simulink model "Vespula_HIiLo_Control"  (R2025b)
settings: Solver=VariableStepAuto  StartTime=0.0  StopTime=30.0  RelTol=1e-3
InitFcn:
  | load('FuelPropsData.mat')
libraries: fl_lib x33, nesl_utility x27, SimscapeFluids_lib x10
(part 1 of 3)
settings Model: Creator=mbdal  LastModifiedBy=25han
settings SolverCC: MaxConsecutiveMinStep=100  ZeroCrossAlgorithm=Adaptive
settings OptimizationCC: ReuseModelBlockBuffer=off
settings DebuggingCC: IgnoredZcDiagnostic=none
settings RTWCC: GPUComputeCapability=3.5

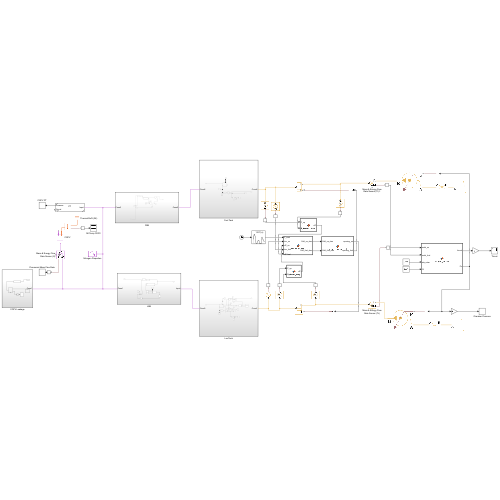
[thumbnail: Simulink's stored preview of the top-level diagram]
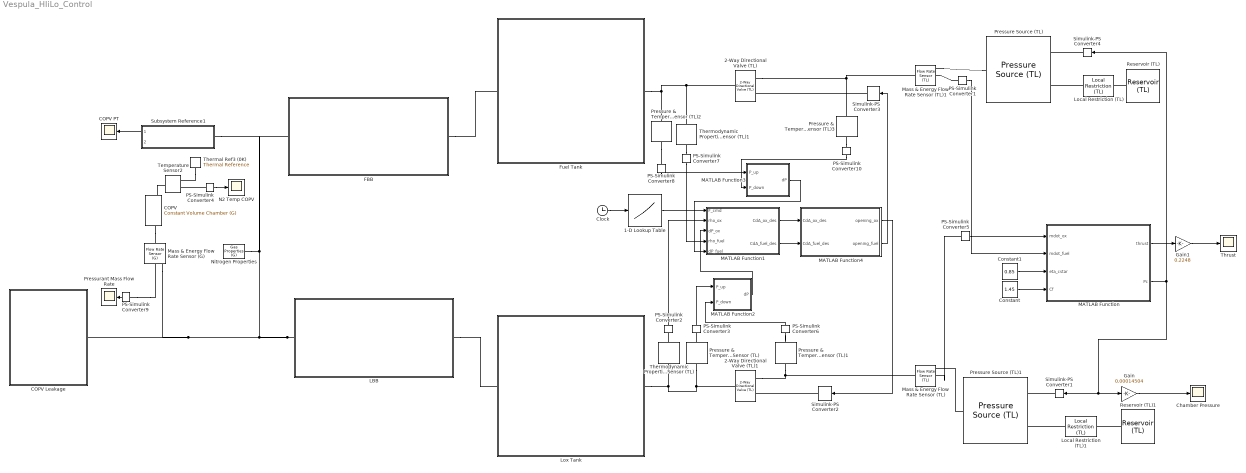
== system Vespula_HIiLo_Control ==
  1-D Lookup Table : Lookup_n-D  NumberOfTableDimensions=1  BreakpointsForDimension1=|  Table=|  InternalRulePriority=Speed  RndMeth=Simplest
      BreakpointsForDimension1=|
      | [0
      | 2.46e-15
      | 4.93e-15
      | 1.31e-14
      | 1.85798e-4
      | 3.71595e-4
      | 1.300583e-3
      | 5.945524e-3
      | 2.917023e-2
      | 1.452937e-1
      | 3.251823e-1
      | 6.176896e-1
      | 1.048884
      | 1.648122
      | 2.452841
      | 3.452841
      | 4.452841
      | 5.452841
      | 6.452841
      | 7.452841
      | 8.452841
      | 9.452841
      | 10.45284
      | 11.45284
      | 12.45284
      | 13.45284
      | 14.45284
      | 15.45284
      | 16.26888
      | 17.26888
      | 18.26888
      | 19.26888
      | 20.26888
      | 21.26888
      | 21.82014
      | 22.37140
      | 23.10183
      | 24.10183
      | 25.10183
      | 26.10183
      | 27.10183
      | 28.10183
      | 29.10183
      | 29.70287]
      Table=|
      | [1115.929794
      | 1115.929794
      | 1115.929794
      | 1115.929794
      | 1116.015031
      | 1116.100248
      | 1116.526042
      | 1118.647732
      | 1129.075722
      | 1176.888468
      | 1237.984070
      | 1309.087819
      | 1365.657208
      | 1382.500173
      | 1347.869214
      | 1276.732855
      | 1209.886660
      | 1007.359221
      | 890.000000
      | 890.000000
      | 890.000000
      | 890.000000
      | 970.372958
      | 1015.368113
      | 1034.720854
      | 1040.888013
      | 1040.596927
      | 896.870767
      | 890.000000
      | 890.000000
      | 890.000000
      | 890.000000
      | 890.000000
      | 890.000000
      | 1074.062231
      | 1213.486737
      | 1218.338865
      | 1172.384789
      | 1114.978943
      | 1066.195681
      | 1030.043331
      | 1004.841448
      | 987.599936
      | 979.912878]
  2-Way Directional Valve (TL) : SimscapeFluids_lib/Thermal Liquid/Valves & Orifices/Directional Control Valves/2-Way Directional Valve (TL)  valve_spec=fluids.thermal_liquid.valves.directional_control_valves.enum.ValveSpec.Table1DAreaOpening  S_max=1 m  del_S_max=5e-3 m  area_max=1e-4 m^2  area_leak=1e-10 m^2  del_S_TLU=[0 0.3 0.4 0.5 0.6 0.7 0.8 0.9 1.0] m  valve_area_TLU=[1e-9 1.7065e-07 1.0239e-06 3.5836e-06 7.8498e-06 1.4164e-05 2.3038e-05 3.4812e-05 5.0000e-05] m^2  del_S_flow_TLU=[0, .002, .004, .007, .017] m  p_diff_TLU=[.3, .5, .7] MPa  vol_flow_TLU=1e-3 * [1.7e-05, 2e-05, 2.6e-05; .0035, .0045, .0053; .7, .9, 1.06; 1.96, 2.5, 3; 6, 7.7, 9.13] m^3/s  mdot_TLU=[1.7e-05, 2e-05, 2.6e-05; .0035, .0045, .0053; .7, .9, 1.06; 1.96, 2.5, 3; 6, 7.7, 9.13] kg/s  T_ref_in=293.15 K  p_ref_in=0.101325 MPa  Cd=1  Re_c=150  smoothing_factor=0.01  pressure_recovery=false  area=0.01 m^2
      settings: InternalSimscapePortConfiguration="{\"Bottom\":[],\"Left\":[{\"id\":\"A\",\"label\":\"A\",\"type\":\"foundation.thermal_liquid.thermal_liquid\"}],\"Right\":[{\"id\":\"S\",\"label\":\"S\",\"type\":\"input\"},{\"id\":\"B\",\"label\":\"B\",\"type\":\"foundation.thermal_liquid.thermal_liquid\"}],\"Top\":[]}"
  2-Way Directional Valve (TL)1 : SimscapeFluids_lib/Thermal Liquid/Valves & Orifices/Directional Control Valves/2-Way Directional Valve (TL)  valve_spec=fluids.thermal_liquid.valves.directional_control_valves.enum.ValveSpec.Table1DAreaOpening  S_max=1 m  del_S_max=5e-3 m  area_max=1e-4 m^2  area_leak=1e-10 m^2  del_S_TLU=[0 0.3 0.4 0.5 0.6 0.7 0.8 0.9 1.0] m  valve_area_TLU=[1e-9 1.7065e-07 1.0239e-06 3.5836e-06 7.8498e-06 1.4164e-05 2.3038e-05 3.4812e-05 5.0000e-05] m^2  del_S_flow_TLU=[0, .002, .004, .007, .017] m  p_diff_TLU=[.3, .5, .7] MPa  vol_flow_TLU=1e-3 * [1.7e-05, 2e-05, 2.6e-05; .0035, .0045, .0053; .7, .9, 1.06; 1.96, 2.5, 3; 6, 7.7, 9.13] m^3/s  mdot_TLU=[1.7e-05, 2e-05, 2.6e-05; .0035, .0045, .0053; .7, .9, 1.06; 1.96, 2.5, 3; 6, 7.7, 9.13] kg/s  T_ref_in=293.15 K  p_ref_in=0.101325 MPa  Cd=1  Re_c=150  smoothing_factor=0.01  pressure_recovery=false  area=0.01 m^2
      settings: InternalSimscapePortConfiguration="{\"Bottom\":[],\"Left\":[{\"id\":\"A\",\"label\":\"A\",\"type\":\"foundation.thermal_liquid.thermal_liquid\"}],\"Right\":[{\"id\":\"S\",\"label\":\"S\",\"type\":\"input\"},{\"id\":\"B\",\"label\":\"B\",\"type\":\"foundation.thermal_liquid.thermal_liquid\"}],\"Top\":[]}"
  COPV : fl_lib/Gas/Elements/Constant Volume Chamber (G)  volume=18 l  num_ports=foundation.enum.num_ports.two  area_A=0.01 m^2  area_B=0.8 in^2  area_C=0.01 m^2  area_D=0.01 m^2  p_I_specify=on  p_I_priority=Low  p_I=4500 psi  p_I_nominal_specify=off  p_I_nominal_value=1  p_I_nominal_unit=MPa  T_I_specify=on  T_I_priority=Low  T_I=60 degF  T_I_nominal_specify=off  T_I_nominal_value=1  T_I_nominal_unit=K  rho_I_specify=off  rho_I_priority=None  rho_I=1.2 kg/m^3  rho_I_nominal_specify=off  rho_I_nominal_value=1  rho_I_nominal_unit=kg/m^3
      settings: InternalSimscapePortConfiguration="{\"Bottom\":[],\"Left\":[{\"id\":\"A\",\"label\":\"A\",\"type\":\"foundation.gas.gas\"},{\"id\":\"H\",\"label\":\"H\",\"type\":\"foundation.thermal.thermal\"}],\"Right\":[{\"id\":\"B\",\"label\":\"B\",\"type\":\"foundation.gas.gas\"}],\"Top\":[]}"
  COPV Leakage : Subsystem
  COPV PT : Scope
      settings: ActiveDisplayYMinimum=1666.95319727996  ActiveDisplayYMaximum=5313.5498863404391  DataLoggingVariableName=ScopeData4  DataLoggingSaveFormat=Array
  Chamber Pressure : Scope
      settings: ActiveDisplayYMinimum=-162.39251881911565  ActiveDisplayYMaximum=515.77790198606317  DataLoggingVariableName=ScopeData22
  Clock : Clock
  Constant : Constant  Value=1.45
  Constant1 : Constant  Value=0.85
  FBB : Subsystem
  Fuel Tank : Subsystem
  Gain : Gain  Gain=0.00014504
  Gain1 : Gain  Gain=0.2248
  LBB : Subsystem
  Local Restriction (TL) : fl_lib/Thermal Liquid/Elements/Local Restriction (TL)  restriction_type=foundation.enum.restriction_type.fixed  restriction_area=0.001 m^2  min_area=1e-10 m^2  max_area=0.005 m^2  area=0.01 m^2  Cd=0.64  Re_c=150  pressure_recovery=true
  Local Restriction (TL)1 : fl_lib/Thermal Liquid/Elements/Local Restriction (TL)  restriction_type=foundation.enum.restriction_type.fixed  restriction_area=0.001 m^2  min_area=1e-10 m^2  max_area=0.005 m^2  area=0.01 m^2  Cd=0.64  Re_c=150  pressure_recovery=true
  Lox Tank : Subsystem
  MATLAB Function : MATLAB Function  TreatAsAtomicUnit=on
  MATLAB Function1 : MATLAB Function  TreatAsAtomicUnit=on
  MATLAB Function2 : MATLAB Function  TreatAsAtomicUnit=on
  MATLAB Function3 : MATLAB Function  TreatAsAtomicUnit=on
  MATLAB Function4 : MATLAB Function  TreatAsAtomicUnit=on
  Mass & Energy Flow Rate Sensor (G) : fl_lib/Gas/Sensors/Flow Rate Sensor (G)  mass_flow_measure=true  volumetric_flow_measure=false  volumetric_flow_conditions=foundation.enum.volumetric_flow_conditions.actual  p_std=0.101325 MPa  T_std=20 degC  energy_flow_measure=true
      settings: InternalSimscapePortConfiguration="{\"Bottom\":[{\"id\":\"PHI\",\"label\":\"φ\",\"type\":\"output\"}],\"Left\":[{\"id\":\"A\",\"label\":\"A\",\"type\":\"foundation.gas.gas\"}],\"Right\":[{\"id\":\"B\",\"label\":\"B\",\"type\":\"foundation.gas.gas\"},{\"id\":\"M\",\"label\":\"M\",\"type\":\"output\"}],\"Top\":[]}"
  Mass & Energy Flow Rate Sensor (TL) : fl_lib/Thermal Liquid/Sensors/Flow Rate Sensor (TL)  mass_flow_measure=true  volumetric_flow_measure=false  energy_flow_measure=true
      settings: InternalSimscapePortConfiguration="{\"Bottom\":[{\"id\":\"PHI\",\"label\":\"φ\",\"type\":\"output\"}],\"Left\":[{\"id\":\"A\",\"label\":\"A\",\"type\":\"foundation.thermal_liquid.thermal_liquid\"}],\"Right\":[{\"id\":\"B\",\"label\":\"B\",\"type\":\"foundation.thermal_liquid.thermal_liquid\"},{\"id\":\"M\",\"label\":\"M\",\"type\":\"output\"}],\"Top\":[]}"
  Mass & Energy Flow Rate Sensor (TL)1 : fl_lib/Thermal Liquid/Sensors/Flow Rate Sensor (TL)  mass_flow_measure=true  volumetric_flow_measure=false  energy_flow_measure=true
      settings: InternalSimscapePortConfiguration="{\"Bottom\":[{\"id\":\"PHI\",\"label\":\"φ\",\"type\":\"output\"}],\"Left\":[{\"id\":\"A\",\"label\":\"A\",\"type\":\"foundation.thermal_liquid.thermal_liquid\"}],\"Right\":[{\"id\":\"B\",\"label\":\"B\",\"type\":\"foundation.thermal_liquid.thermal_liquid\"},{\"id\":\"M\",\"label\":\"M\",\"type\":\"output\"}],\"Top\":[]}"
  N2 Temp COPV : Scope
      settings: ActiveDisplayYMinimum=266.75436250244837  ActiveDisplayYMaximum=294.5410897859407  DataLoggingVariableName=ScopeData11
  Nitrogen Properties : fl_lib/Gas/Utilities/Gas Properties (G)  gas_spec=foundation.enum.gas_spec.real_gas  R=0.297 kJ/(K*kg)  Z=1  T_ref=293.0 K  h_ref=425.45 kJ/kg  cp_ref=1.1305 kJ/(K*kg)  mu_ref=24.664 s*uPa  k_ref=24.664 W/(m*K)  T_TLU1=[150 : 10 : 200, 250 : 50 : 1000, 1500, 2000]' K  h_TLU1=[275.264783730547; 285.377054177734; 295.474578903607; 305.560871069627; 315.638490783961; 325.709373787179; 376.008033649461; 426.297784741196; 476.678788323875; 527.253890684429; 578.12722735187; 629.395040865183; 681.137690131207; 733.415442873049; 786.267894376777; 839.715851152006; 893.764459999509; 948.406676876931; 1003.62653219711; 1059.40193232821; 1115.70691941005; 1172.51341226958; 1762.18512007361; 2377.14064127409] kJ/kg  cp_TLU1=[1.01211492398124; 1.01042105529234; 1.00914159006373; 1.00815898273273; 1.00739688341918; 1.00680484569075; 1.00554191216852; 1.00637389921747; 1.0092105862442; 1.01414404435034; 1.02111299587909; 1.02986878923959; 1.04003820504128; 1.05120320041448; 1.06296312852444; 1.07497111709439; 1.08694865668905; 1.0986858495625; 1.11003396604319; 1.12089493621399; 1.13121051694521; 1.14095251451866; 1.21001953144; 1.24628356718428] kJ/(K*kg)  mu_TLU1=[10.3766056544352; 10.9908682444892; 11.5932000841352; 12.1841060353213; 12.764067709023; 13.3335437107148; 16.038149065057; 18.5373404836509; 20.8671495114253; 23.0554226800681; 25.1239717991959; 27.0901379793485; 28.96790749834; 30.7687111230031; 32.5020036481173; 34.17569027566; 35.7964450415303; 37.3699520751368; 38.9010908824946; 40.3940804368247; 41.8525925389218; 43.279841956487; 56.3254722619962; 68.068290080945] s*uPa  k_TLU1=[14.1517155766309; 15.0474512994325; 15.9300520513026; 16.7998749295306; 17.6573089963228; 18.5027588910197; 22.5644026699512; 26.384465676638; 30.0032801168886; 33.4532006033488; 36.7600619429332; 39.9446251241844; 43.0237448740114; 46.0112537033799; 48.9186234516389; 51.7554617696538; 54.5298878921773; 57.2488200454925; 59.9181976996146; 62.5431553064749; 65.128159527924; 67.6771186900213; 91.7815514375552; 114.486299090693] mW/(K*m)  T_TLU2=[ 150 160 170 180 190 200 250 300 350 400 450 500 550 600 650 700 750 800 850 900 950 1000 1500 2000 ] K  p_TLU2=[ 0.001 0.005 0.01 0.02 0.03 0.04 0.05 0.06 0.07 0.08 0.09 0.1 0.12 0.15 0.2 0.5 1 2 5 10 15 20 25 30 35 ] MPa  rho_TLU2=|  s_TLU2=|  h_TLU2=|  cp_TLU2=|  mu_TLU2=|  k_TLU2=|  beta_TLU2=|  alpha_TLU2=|  T_min_perfect=1 K  T_max_perfect=inf K  p_min_perfect=1 Pa  p_max_perfect=inf MPa  T_range_flag=foundation.enum.T_range_G.from_props  T_min_semiperfect=150 K  T_max_semiperfect=2000 K  p_min_semiperfect=1 Pa  p_max_semiperfect=inf MPa  pT_region_flag=foundation.enum.pT_region_G.from_props  pT_validity_TLU2=ones(24, 20)  T_min_real=150 K  T_max_real=2000 K  p_min_real=0.001 MPa  p_max_real=10 MPa  p_atm=0.101325 MPa  properties_range_check=simscape.enum.assert.action.error  Mach_rev=0.001
      rho_TLU2=|
      | [
      |   0.0224628 0.11234 0.224745 0.449748 0.675012 0.900536 1.12632 1.35237 1.57868 1.80525 2.03209 2.25919 2.71419 3.39869 4.54491 11.5684 23.876 51.1797 168.905 419.166 512.081 561.75 596.092 622.603 644.346
      |   0.0210587 0.105313 0.210675 0.421548 0.632619 0.843889 1.05536 1.26702 1.47889 1.69096 1.90322 2.11569 2.54123 3.18105 4.25149 10.7835 22.111 46.6336 140.444 344.171 458.334 518.814 559.223 589.665 614.197
      |   0.0198197 0.0991139 0.198266 0.396684 0.595255 0.793978 0.992854 1.19188 1.39107 1.5904 1.78989 1.98953 2.38928 2.99007 3.99448 10.104 20.6157 42.9807 122.906 287.979 407.95 477.264 523.326 557.57 584.838
      |   0.0187185 0.0936044 0.187238 0.374595 0.56207 0.749663 0.937375 1.12521 1.31315 1.50122 1.68941 1.87772 2.25469 2.82104 3.76735 9.50897 19.3276 39.9514 110.475 248.744 363.904 438.437 489.087 526.714 556.514
      |   0.0177332 0.0886754 0.177374 0.35484 0.532399 0.71005 0.887794 1.06563 1.24356 1.42158 1.59969 1.7779 2.13459 2.67033 3.56509 8.98291 18.2034 37.3816 100.976 220.597 327.193 403.291 457.086 497.451 529.453
      |   0.0168465 0.0842398 0.168498 0.337068 0.50571 0.674425 0.843213 1.01207 1.18101 1.35001 1.51909 1.68824 2.02676 2.53508 3.38374 8.51404 17.2116 35.1639 93.3657 199.439 297.167 372.228 427.691 470.049 503.836
      |   0.013477 0.0673872 0.13478 0.269581 0.404403 0.539247 0.674112 0.808998 0.943905 1.07883 1.21378 1.34875 1.61876 2.02392 2.69962 6.76469 13.5801 27.3519 69.5435 140.592 208.08 268.096 319.417 362.758 399.494
      |   0.0112308 0.0561543 0.11231 0.224623 0.336941 0.449263 0.561589 0.673919 0.786253 0.898591 1.01093 1.12328 1.34798 1.68507 2.24695 5.6202 11.2488 22.5234 56.3445 111.725 164.239 212.537 256.035 294.781 329.184
      |   0.00962635 0.0481315 0.0962625 0.192523 0.288781 0.385036 0.48129 0.577541 0.67379 0.770036 0.86628 0.962522 1.155 1.44369 1.92481 4.81016 9.61356 19.1957 47.6684 93.741 137.378 178.031 215.461 249.68 280.866
      |   0.00842305 0.0421148 0.0842284 0.168452 0.252671 0.336886 0.421096 0.505301 0.589502 0.673698 0.757889 0.842076 1.01043 1.26294 1.68369 4.20567 8.39918 16.7473 41.4399 81.1856 118.842 154.174 187.094 217.632 245.899
      |   0.00748715 0.0374352 0.0748691 0.149733 0.224591 0.299444 0.374292 0.449134 0.523971 0.598803 0.673629 0.74845 0.898076 1.12247 1.49637 3.73687 7.46006 14.8641 36.7155 71.8128 105.105 136.495 165.968 193.564 219.367
      |   0.00673843 0.0336916 0.0673819 0.134758 0.20213 0.269495 0.336856 0.404211 0.47156 0.538905 0.606244 0.673577 0.808228 1.01016 1.34662 3.36249 6.71139 13.3677 32.9929 64.4976 94.4306 122.764 149.512 174.722 198.464
      |   0.00612584 0.0306287 0.0612561 0.122507 0.183753 0.244994 0.30623 0.36746 0.428686 0.489906 0.551121 0.612331 0.734736 0.918305 1.22415 3.05653 6.10019 12.1485 29.9758 58.6032 85.8531 111.73 136.264 159.502 181.505
      |   0.00561536 0.0280763 0.0561514 0.112298 0.16844 0.224577 0.28071 0.336837 0.39296 0.449078 0.505192 0.561301 0.673504 0.841773 1.12213 2.80175 5.59158 11.1353 27.4767 53.7382 78.7843 102.636 125.328 146.908 167.426
      |   0.00518341 0.0259166 0.0518321 0.10366 0.155483 0.207302 0.259117 0.310927 0.362733 0.414535 0.466332 0.518125 0.621697 0.777024 1.03581 2.58626 5.1616 10.2795 25.37 49.6461 72.8431 94.9893 116.122 136.283 155.52
      |   0.00481316 0.0240654 0.0481298 0.0962557 0.144378 0.192495 0.240609 0.288719 0.336825 0.384927 0.433025 0.481119 0.577295 0.721529 0.96184 2.40161 4.79327 9.54671 23.5687 46.1513 67.7704 88.4569 108.247 127.18 145.298
      |   0.00449229 0.0224611 0.0449212 0.0898388 0.134753 0.179663 0.22457 0.269473 0.314372 0.359268 0.40416 0.449049 0.538815 0.673437 0.897734 2.24161 4.47416 8.91208 22.0097 43.1286 63.3825 82.8028 101.424 119.282 136.413
      |   0.00421152 0.0210573 0.0421137 0.0842241 0.126331 0.168435 0.210535 0.252632 0.294726 0.336817 0.378904 0.420988 0.505146 0.631358 0.841645 2.10163 4.195 8.357 20.6467 40.4863 59.5457 77.8551 95.4466 112.353 128.607
      |   0.00396378 0.0198186 0.0396365 0.0792699 0.1189 0.158528 0.198152 0.237773 0.277392 0.317007 0.356619 0.396229 0.475438 0.59423 0.792155 1.97812 3.9487 7.86733 19.4444 38.1554 56.1594 73.485 90.1619 106.22 121.688
      |   0.00374357 0.0187176 0.0374345 0.0748662 0.112295 0.149721 0.187145 0.224565 0.261983 0.299398 0.336811 0.37422 0.449031 0.561227 0.748164 1.86834 3.72979 7.43208 18.3758 36.083 53.1469 69.5942 85.4522 100.748 115.507
      |   0.00354654 0.0177325 0.0354643 0.070926 0.106385 0.141842 0.177296 0.212748 0.248197 0.283643 0.319087 0.354529 0.425404 0.531698 0.708804 1.77011 3.53391 7.04264 17.4195 34.2275 50.4481 66.1058 81.2256 95.8317 109.948
      |   0.00336922 0.0168458 0.0336911 0.0673799 0.101066 0.13475 0.168432 0.202112 0.235789 0.269464 0.303136 0.336806 0.40414 0.505122 0.67338 1.68171 3.35761 6.69211 16.5585 32.5562 48.0155 62.959 77.4094 91.3888 104.918
      |   0.00224615 0.0112306 0.022461 0.0449208 0.0673795 0.0898371 0.112294 0.134749 0.157203 0.179656 0.202108 0.224559 0.269457 0.336796 0.449005 1.12167 2.24054 4.46991 11.0918 21.9124 32.4719 42.7798 52.8458 62.6786 72.2871
      |   0.00168461 0.00842299 0.0168458 0.033691 0.0505355 0.0673794 0.0842226 0.101065 0.117907 0.134748 0.151589 0.168429 0.202107 0.25262 0.336794 0.841502 1.6814 3.35638 8.34329 16.5303 24.5658 32.4546 40.2011 47.8097 55.2845
      | ] kg/m^3
      s_TLU2=|
      | [
      |   7.49285 7.01501 6.8091 6.603 6.48229 6.39654 6.32994 6.27546 6.22933 6.18933 6.154 6.12236 6.0675 6.00016 5.9129 5.62948 5.40371 5.15375 4.7005 4.22784 4.07775 3.99456 3.93507 3.88788 3.84829
      |   7.55991 7.08209 6.87621 6.67017 6.54951 6.46381 6.39727 6.34284 6.29678 6.25683 6.22156 6.18997 6.13523 6.06805 5.98109 5.69949 5.4771 5.23565 4.83347 4.40808 4.22227 4.12381 4.05631 4.00418 3.96125
      |   7.6229 7.1451 6.93924 6.73324 6.61263 6.52698 6.46048 6.4061 6.36008 6.32017 6.28495 6.2534 6.19875 6.13171 6.04497 5.76478 5.54497 5.30962 4.93669 4.55875 4.35631 4.24459 4.1695 4.1126 4.06642
      |   7.68229 7.20451 6.99867 6.7927 6.67213 6.58651 6.52005 6.4657 6.41971 6.37985 6.34465 6.31315 6.25857 6.19163 6.10508 5.82601 5.60821 5.37744 5.02371 4.6809 4.47723 4.35635 4.27486 4.21367 4.16448
      |   7.73847 7.2607 7.05487 6.84894 6.72839 6.6428 6.57637 6.52205 6.47609 6.43626 6.40109 6.36962 6.31509 6.24825 6.16184 5.88369 5.66748 5.44026 5.10015 4.78242 4.58443 4.45885 4.37256 4.30779 4.25597
      |   7.79177 7.31401 7.10819 6.90228 6.78176 6.69619 6.62978 6.57549 6.52956 6.48974 6.45461 6.42315 6.36868 6.30191 6.21562 5.93821 5.72331 5.4989 5.16896 4.86953 4.67917 4.55232 4.46291 4.39539 4.34139
      |   8.02365 7.54592 7.34014 7.1343 7.01386 6.92836 6.86203 6.80781 6.76195 6.72222 6.68715 6.65577 6.60145 6.5349 6.44899 6.17388 5.96289 5.74667 5.44372 5.18996 5.02917 4.9123 4.82264 4.75128 4.69272
      |   8.21316 7.73544 7.52968 7.32388 7.20347 7.11802 7.05172 6.99754 6.95172 6.91202 6.87699 6.84565 6.7914 6.72497 6.63924 6.36524 6.15613 5.94369 5.65221 5.41654 5.27019 5.16301 5.0789 5.01026 4.95271
      |   8.37353 7.89582 7.69007 7.48429 7.3639 7.27847 7.21219 7.15803 7.11223 7.07255 7.03754 7.00622 6.95202 6.88564 6.80002 6.52665 6.31857 6.10821 5.82285 5.59656 5.45806 5.35694 5.27722 5.21162 5.15607
      |   8.51273 8.03503 7.82928 7.62352 7.50314 7.41772 7.35146 7.29731 7.25152 7.21185 7.17686 7.14555 7.09137 7.02504 6.93948 6.66649 6.45906 6.24996 5.96826 5.74757 5.61385 5.51664 5.44002 5.3768 5.32307
      |   8.63597 8.15828 7.95253 7.74678 7.62641 7.541 7.47474 7.4206 7.37482 7.33516 7.30018 7.26888 7.21472 7.14841 7.06289 6.79016 6.58314 6.37487 6.09556 5.87849 5.74792 5.65337 5.57895 5.51753 5.46526
      |   8.74684 8.26914 8.06341 7.85766 7.73729 7.65189 7.58564 7.5315 7.48573 7.44608 7.4111 7.37981 7.32565 7.25936 7.17388 6.90131 6.69459 6.48688 6.20922 5.99465 5.86627 5.7736 5.70079 5.64074 5.58961
      |   8.84788 8.37018 8.16445 7.9587 7.83834 7.75294 7.68669 7.63256 7.5868 7.54715 7.51217 7.48089 7.42674 7.36046 7.275 7.00256 6.79604 6.58874 6.31225 6.09947 5.97268 5.88141 5.80981 5.7508 5.70057
      |   8.94094 8.46325 8.25751 8.05177 7.93141 7.84602 7.77977 7.72565 7.67988 7.64024 7.60526 7.57398 7.51984 7.45357 7.36812 7.09578 6.88941 6.68241 6.40679 6.19534 6.06974 5.97952 5.90885 5.85065 5.80114
      |   9.02741 8.54972 8.34398 8.13824 8.01789 7.93249 7.86625 7.81213 7.76636 7.72672 7.69175 7.66047 7.60634 7.54007 7.45464 7.18236 6.97611 6.76934 6.49438 6.28395 6.15926 6.06985 5.99991 5.94236 5.89343
      |   9.10832 8.63063 8.4249 8.21916 8.09881 8.01341 7.94717 7.89305 7.84729 7.80765 7.77268 7.7414 7.68727 7.62101 7.53558 7.26336 7.0572 6.85061 6.57616 6.36652 6.24254 6.15379 6.08442 6.0274 5.97893
      |   9.18448 8.70679 8.50105 8.29532 8.17497 8.08957 8.02334 7.96922 7.92346 7.88382 7.84885 7.81757 7.76344 7.69719 7.61177 7.33959 7.1335 6.92705 6.653 6.44399 6.32058 6.23234 6.16345 6.10685 6.05877
      |   9.2565 8.77881 8.57308 8.36734 8.247 8.1616 8.09537 8.04125 7.99549 7.95585 7.92089 7.88961 7.83548 7.76923 7.68382 7.41167 7.20564 6.9993 6.72558 6.51706 6.39412 6.3063 6.23779 6.18154 6.13378
      |   9.32489 8.8472 8.64147 8.43573 8.31539 8.22999 8.16376 8.10964 8.06388 8.02424 7.98928 7.958 7.90388 7.83763 7.75222 7.48011 7.27412 7.06787 6.79441 6.58631 6.46374 6.37627 6.30808 6.25212 6.20463
      |   9.39004 8.91235 8.70662 8.50088 8.38054 8.29515 8.22891 8.17479 8.12904 8.0894 8.05444 8.02316 7.96904 7.9028 7.81739 7.54529 7.33934 7.13317 6.85993 6.65216 6.52991 6.44273 6.3748 6.31909 6.27183
      |   9.45228 8.97459 8.76886 8.56313 8.44278 8.35739 8.29116 8.23704 8.19128 8.15165 8.11668 8.08541 8.03129 7.96504 7.87964 7.60757 7.40165 7.19554 6.92247 6.71499 6.593 6.50606 6.43836 6.38285 6.33579
      |   9.51188 9.03419 8.82846 8.62273 8.50238 8.41699 8.35076 8.29664 8.25089 8.21125 8.17629 8.14502 8.0909 8.02466 7.93925 7.6672 7.4613 7.25525 6.98233 6.77509 6.65331 6.56658 6.49907 6.44374 6.39684
      |   10.0013 9.52364 9.31791 9.11218 8.99183 8.90645 8.84022 8.7861 8.74035 8.70072 8.66576 8.63449 8.58037 8.51414 8.42875 8.15676 7.95099 7.74518 7.47298 7.26687 7.14616 7.06043 6.99387 6.93944 6.89338
      |   10.3653 9.88756 9.68184 9.47611 9.35576 9.27038 9.20415 9.15003 9.10428 9.06465 9.02969 8.99842 8.9443 8.87807 8.79269 8.52073 8.31499 8.10925 7.83725 7.63147 7.51108 7.42564 7.35937 7.30522 7.25943
      | ] kJ/(K*kg)
      h_TLU2=|
      | [
      |   155.532 155.5 155.459 155.379 155.298 155.217 155.136 155.055 154.974 154.893 154.811 154.73 154.567 154.323 153.913 151.418 147.102 137.79 102.023 48.5204 36.6348 33.4423 33.1456 34.2668 36.2186
      |   165.923 165.894 165.858 165.786 165.713 165.641 165.569 165.496 165.424 165.352 165.279 165.206 165.061 164.843 164.478 162.264 158.473 150.476 122.598 76.439 59.0269 53.4698 51.9312 52.2875 53.7211
      |   176.314 176.288 176.255 176.19 176.125 176.06 175.995 175.93 175.865 175.8 175.735 175.669 175.539 175.343 175.016 173.035 169.668 162.676 139.613 101.272 81.1345 73.3902 70.6014 70.1706 71.0675
      |   186.704 186.681 186.651 186.593 186.534 186.475 186.416 186.357 186.299 186.24 186.181 186.122 186.004 185.827 185.531 183.747 180.731 174.539 154.83 122.628 102.284 92.9408 89.0315 87.8503 88.2213
      |   197.095 197.074 197.047 196.994 196.94 196.887 196.833 196.78 196.726 196.673 196.619 196.566 196.459 196.298 196.03 194.414 191.693 186.157 168.964 141.394 122.104 111.896 107.1 105.258 105.143
      |   207.486 207.467 207.442 207.393 207.345 207.296 207.247 207.198 207.15 207.101 207.052 207.003 206.906 206.759 206.515 205.044 202.577 197.589 182.377 158.372 140.569 130.115 124.713 122.334 121.795
      |   259.444 259.431 259.415 259.382 259.35 259.318 259.286 259.254 259.222 259.189 259.157 259.125 259.061 258.964 258.804 257.841 256.241 253.066 243.814 229.877 218.643 210.476 205.084 201.897 200.368
      |   311.415 311.406 311.395 311.373 311.351 311.329 311.307 311.285 311.263 311.241 311.218 311.196 311.152 311.086 310.976 310.317 309.227 307.082 300.952 291.933 284.632 279.109 275.243 272.811 271.57
      |   363.432 363.426 363.419 363.403 363.388 363.373 363.357 363.342 363.326 363.311 363.296 363.28 363.25 363.204 363.127 362.67 361.917 360.442 356.283 350.292 345.523 341.959 339.514 338.066 337.479
      |   415.558 415.553 415.548 415.538 415.527 415.516 415.506 415.495 415.485 415.474 415.464 415.453 415.432 415.401 415.348 415.034 414.519 413.516 410.728 406.822 403.837 401.733 400.444 399.889 399.982
      |   467.879 467.876 467.872 467.865 467.858 467.851 467.844 467.837 467.83 467.823 467.816 467.809 467.796 467.775 467.74 467.533 467.195 466.542 464.764 462.396 460.743 459.765 459.409 459.616 460.326
      |   520.495 520.493 520.491 520.487 520.482 520.478 520.474 520.47 520.466 520.461 520.457 520.453 520.445 520.432 520.411 520.287 520.086 519.702 518.7 517.514 516.9 516.817 517.223 518.074 519.326
      |   573.502 573.502 573.501 573.499 573.497 573.494 573.492 573.49 573.488 573.486 573.484 573.482 573.478 573.472 573.462 573.404 573.311 573.14 572.754 572.507 572.724 573.37 574.409 575.808 577.531
      |   626.984 626.984 626.983 626.983 626.983 626.983 626.982 626.982 626.982 626.982 626.981 626.981 626.981 626.98 626.979 626.973 626.968 626.97 627.082 627.599 628.499 629.749 631.322 633.189 635.323
      |   681.001 681.001 681.002 681.003 681.004 681.006 681.007 681.008 681.009 681.01 681.012 681.013 681.015 681.019 681.025 681.064 681.13 681.275 681.799 682.948 684.417 686.177 688.204 690.475 692.969
      |   735.596 735.597 735.598 735.6 735.603 735.605 735.608 735.61 735.612 735.615 735.617 735.62 735.625 735.632 735.645 735.719 735.847 736.111 736.979 738.661 740.611 742.806 745.224 747.848 750.658
      |   790.791 790.792 790.794 790.797 790.801 790.804 790.808 790.811 790.815 790.818 790.822 790.825 790.832 790.843 790.86 790.966 791.145 791.51 792.671 794.806 797.169 799.738 802.497 805.428 808.519
      |   846.594 846.595 846.598 846.602 846.606 846.611 846.615 846.62 846.624 846.628 846.633 846.637 846.646 846.659 846.681 846.813 847.036 847.488 848.9 851.425 854.144 857.039 860.096 863.299 866.638
      |   902.999 903.001 903.004 903.009 903.014 903.019 903.024 903.029 903.034 903.04 903.045 903.05 903.06 903.076 903.101 903.257 903.517 904.044 905.674 908.536 911.566 914.748 918.067 921.512 925.073
      |   959.992 959.994 959.997 960.003 960.009 960.015 960.02 960.026 960.032 960.038 960.044 960.05 960.061 960.079 960.108 960.283 960.577 961.169 962.988 966.146 969.45 972.883 976.435 980.096 983.855
      |   1017.55 1017.55 1017.56 1017.56 1017.57 1017.58 1017.58 1017.59 1017.6 1017.6 1017.61 1017.62 1017.63 1017.65 1017.68 1017.87 1018.2 1018.84 1020.83 1024.25 1027.79 1031.45 1035.21 1039.06 1043
      |   1075.65 1075.66 1075.66 1075.67 1075.67 1075.68 1075.69 1075.7 1075.7 1075.71 1075.72 1075.72 1075.74 1075.76 1075.79 1076 1076.35 1077.05 1079.18 1082.83 1086.59 1090.45 1094.39 1098.42 1102.52
      |   1680.51 1680.51 1680.52 1680.53 1680.54 1680.55 1680.56 1680.57 1680.58 1680.59 1680.6 1680.61 1680.63 1680.66 1680.71 1681 1681.5 1682.49 1685.48 1690.48 1695.51 1700.57 1705.64 1710.74 1715.85
      |   2313.5 2313.51 2313.51 2313.52 2313.54 2313.55 2313.56 2313.57 2313.58 2313.59 2313.6 2313.61 2313.64 2313.67 2313.72 2314.06 2314.61 2315.72 2319.06 2324.62 2330.19 2335.76 2341.33 2346.9 2352.47
      | ] kJ/kg
      cp_TLU2=|
      | [
      |   1.03907 1.03945 1.03991 1.04085 1.04179 1.04273 1.04367 1.04462 1.04557 1.04652 1.04747 1.04843 1.05035 1.05326 1.05816 1.08921 1.14798 1.30032 2.36534 2.85375 2.22971 2.00006 1.88069 1.80707 1.75703
      |   1.03907 1.03939 1.03978 1.04056 1.04135 1.04214 1.04293 1.04372 1.04451 1.04531 1.0461 1.0469 1.04851 1.05093 1.055 1.08049 1.12736 1.24112 1.83366 2.668 2.23733 2.00169 1.87475 1.7962 1.743
      |   1.03907 1.03934 1.03967 1.04034 1.04101 1.04168 1.04235 1.04302 1.0437 1.04437 1.04505 1.04572 1.04708 1.04913 1.05257 1.07389 1.11228 1.20129 1.59489 2.29746 2.17231 1.97785 1.85717 1.7793 1.72567
      |   1.03908 1.03931 1.0396 1.04017 1.04074 1.04132 1.0419 1.04247 1.04305 1.04363 1.04421 1.04479 1.04596 1.04771 1.05065 1.06877 1.10087 1.17286 1.45963 1.99046 2.05138 1.92842 1.82677 1.75546 1.70442
      |   1.03909 1.03929 1.03954 1.04004 1.04053 1.04103 1.04154 1.04204 1.04254 1.04304 1.04354 1.04405 1.04506 1.04658 1.04912 1.06471 1.09199 1.15168 1.37295 1.77628 1.91255 1.86022 1.78535 1.72504 1.67924
      |   1.0391 1.03927 1.03949 1.03993 1.04037 1.04081 1.04124 1.04168 1.04212 1.04256 1.043 1.04344 1.04433 1.04565 1.04788 1.06144 1.08495 1.1354 1.31295 1.62808 1.78336 1.78282 1.73642 1.6895 1.65071
      |   1.03923 1.03933 1.03946 1.03971 1.03996 1.04021 1.04046 1.04071 1.04096 1.04121 1.04146 1.04172 1.04222 1.04297 1.04423 1.05184 1.06467 1.09087 1.17213 1.30277 1.40326 1.46237 1.4886 1.49535 1.49225
      |   1.03974 1.0398 1.03988 1.04004 1.0402 1.04037 1.04053 1.04069 1.04085 1.04101 1.04117 1.04133 1.04166 1.04214 1.04295 1.04781 1.05591 1.07214 1.12034 1.19493 1.25646 1.30206 1.33294 1.35234 1.36369
      |   1.04117 1.04121 1.04127 1.04138 1.04149 1.04161 1.04172 1.04183 1.04194 1.04206 1.04217 1.04228 1.0425 1.04284 1.0434 1.04676 1.05234 1.06341 1.09571 1.14502 1.18681 1.22032 1.24603 1.26514 1.279
      |   1.04414 1.04417 1.04421 1.04429 1.04438 1.04446 1.04454 1.04462 1.0447 1.04479 1.04487 1.04495 1.04511 1.04536 1.04577 1.04822 1.05229 1.06032 1.08358 1.11895 1.14943 1.17486 1.19555 1.2121 1.22517
      |   1.04903 1.04906 1.04909 1.04915 1.04922 1.04928 1.04934 1.0494 1.04947 1.04953 1.04959 1.04965 1.04978 1.04996 1.05028 1.05214 1.05523 1.06132 1.07888 1.10561 1.12893 1.14888 1.16567 1.17967 1.19126
      |   1.05594 1.05595 1.05598 1.05603 1.05608 1.05613 1.05618 1.05622 1.05627 1.05632 1.05637 1.05642 1.05652 1.05666 1.05691 1.05837 1.06079 1.06555 1.07928 1.10022 1.11869 1.13475 1.1486 1.16045 1.17055
      |   1.06465 1.06466 1.06468 1.06472 1.06476 1.0648 1.06484 1.06488 1.06492 1.06496 1.065 1.06504 1.06511 1.06523 1.06543 1.0666 1.06854 1.07236 1.08338 1.10023 1.11522 1.12844 1.14002 1.15012 1.15891
      |   1.07481 1.07482 1.07484 1.07487 1.0749 1.07494 1.07497 1.075 1.07503 1.07506 1.0751 1.07513 1.07519 1.07529 1.07545 1.07641 1.078 1.08112 1.09014 1.10398 1.1164 1.12746 1.13728 1.14596 1.15364
      |   1.08601 1.08602 1.08604 1.08606 1.08609 1.08612 1.08614 1.08617 1.0862 1.08622 1.08625 1.08628 1.08633 1.08641 1.08655 1.08734 1.08866 1.09126 1.09877 1.11033 1.12077 1.13015 1.13857 1.1461 1.15283
      |   1.09785 1.09786 1.09787 1.0979 1.09792 1.09794 1.09796 1.09799 1.09801 1.09803 1.09805 1.09808 1.09812 1.09819 1.0983 1.09897 1.10008 1.10228 1.10861 1.1184 1.12729 1.13534 1.14262 1.1492 1.15514
      |   1.10998 1.10999 1.11 1.11002 1.11004 1.11006 1.11008 1.11009 1.11011 1.11013 1.11015 1.11017 1.11021 1.11027 1.11036 1.11093 1.11188 1.11375 1.11916 1.12754 1.13519 1.14217 1.14852 1.1543 1.15957
      |   1.12212 1.12212 1.12213 1.12215 1.12216 1.12218 1.1222 1.12221 1.12223 1.12225 1.12226 1.12228 1.12231 1.12236 1.12244 1.12294 1.12375 1.12536 1.13002 1.13726 1.14391 1.15 1.15559 1.16071 1.1654
      |   1.13404 1.13405 1.13406 1.13407 1.13408 1.1341 1.13411 1.13413 1.13414 1.13416 1.13417 1.13418 1.13421 1.13426 1.13433 1.13475 1.13546 1.13686 1.14091 1.14722 1.15304 1.1584 1.16334 1.16789 1.17209
      |   1.14561 1.14562 1.14562 1.14563 1.14565 1.14566 1.14567 1.14568 1.1457 1.14571 1.14572 1.14573 1.14576 1.1458 1.14586 1.14623 1.14685 1.14807 1.15162 1.15716 1.16229 1.16703 1.17143 1.17549 1.17927
      |   1.15672 1.15672 1.15673 1.15674 1.15675 1.15676 1.15677 1.15678 1.15679 1.1568 1.15681 1.15682 1.15685 1.15688 1.15693 1.15726 1.15781 1.15888 1.162 1.1669 1.17145 1.17567 1.1796 1.18325 1.18665
      |   1.16729 1.1673 1.1673 1.16731 1.16732 1.16733 1.16734 1.16735 1.16736 1.16737 1.16738 1.16739 1.16741 1.16744 1.16749 1.16778 1.16826 1.16921 1.17198 1.17633 1.18038 1.18416 1.18768 1.19097 1.19405
      |   1.24387 1.24388 1.24388 1.24388 1.24388 1.24389 1.24389 1.2439 1.2439 1.2439 1.24391 1.24391 1.24392 1.24393 1.24394 1.24405 1.24423 1.24457 1.24559 1.24722 1.24878 1.25026 1.25167 1.25302 1.25432
      |   1.28404 1.28404 1.28404 1.28404 1.28404 1.28404 1.28404 1.28405 1.28405 1.28405 1.28405 1.28405 1.28405 1.28406 1.28407 1.28411 1.28419 1.28435 1.28481 1.28556 1.28628 1.28697 1.28764 1.28829 1.28892
      | ] kJ/(K*kg)
      mu_TLU2=|
      | [
      |   10.0483 10.0496 10.0512 10.0543 10.0575 10.0606 10.0638 10.067 10.0702 10.0734 10.0766 10.0799 10.0863 10.0961 10.1125 10.2157 10.4068 10.878 13.7553 27.7398 38.1797 45.4394 51.3594 56.5697 61.3491
      |   10.6388 10.64 10.6414 10.6443 10.6473 10.6502 10.6531 10.656 10.659 10.6619 10.6648 10.6678 10.6737 10.6827 10.6978 10.792 10.9646 11.3792 13.5221 22.4016 32.216 39.5241 45.4004 50.4816 55.0779
      |   11.2177 11.2188 11.2201 11.2228 11.2255 11.2282 11.2309 11.2336 11.2363 11.239 11.2417 11.2444 11.2499 11.2582 11.2721 11.3586 11.516 11.8868 13.6322 19.7468 27.8471 34.8201 40.5657 45.5148 49.9527
      |   11.7854 11.7864 11.7876 11.7901 11.7926 11.7951 11.7976 11.8001 11.8026 11.8051 11.8077 11.8102 11.8153 11.8229 11.8358 11.9158 12.0603 12.3958 13.8828 18.5029 24.9193 31.2005 36.6724 41.4491 45.7299
      |   12.3424 12.3433 12.3444 12.3468 12.3491 12.3514 12.3537 12.3561 12.3584 12.3608 12.3631 12.3655 12.3702 12.3773 12.3893 12.4635 12.597 12.9035 14.2051 17.927 23.0742 28.5235 33.5873 38.1314 42.2384
      |   12.8891 12.8899 12.891 12.8932 12.8954 12.8976 12.8997 12.9019 12.9041 12.9063 12.9085 12.9107 12.9151 12.9218 12.9329 13.0022 13.1261 13.408 14.5685 17.6952 21.9438 26.612 31.1917 35.4462 39.3537
      |   15.4832 15.4839 15.4847 15.4863 15.4879 15.4895 15.4912 15.4928 15.4944 15.4961 15.4977 15.4994 15.5027 15.5076 15.5159 15.5671 15.6575 15.8574 16.615 18.3833 20.6289 23.1295 25.7632 28.4703 31.1925
      |   17.8772 17.8777 17.8783 17.8796 17.8809 17.8822 17.8835 17.8848 17.886 17.8873 17.8886 17.8899 17.8925 17.8964 17.9029 17.9431 18.0133 18.1665 18.7258 19.9613 21.487 23.1843 24.9686 26.8042 28.6793
      |   20.1068 20.1072 20.1078 20.1088 20.1099 20.1109 20.112 20.113 20.1141 20.1151 20.1162 20.1172 20.1193 20.1225 20.1279 20.1605 20.2174 20.3404 20.7797 21.7224 22.8702 24.1507 25.5044 26.896 28.3112
      |   22.1996 22.2 22.2004 22.2013 22.2022 22.2031 22.204 22.2048 22.2057 22.2066 22.2075 22.2084 22.2102 22.2128 22.2173 22.2447 22.2921 22.3941 22.7529 23.5087 24.4213 25.4422 26.5292 27.6523 28.7948
      |   24.1771 24.1774 24.1778 24.1786 24.1793 24.1801 24.1808 24.1816 24.1823 24.1831 24.1839 24.1846 24.1862 24.1884 24.1923 24.2157 24.2562 24.3427 24.6439 25.27 26.0216 26.8642 27.767 28.706 29.6649
      |   26.0563 26.0566 26.0569 26.0576 26.0582 26.0589 26.0595 26.0602 26.0609 26.0615 26.0622 26.0628 26.0642 26.0662 26.0695 26.0899 26.125 26.1998 26.4578 26.9888 27.6234 28.336 29.1033 29.9062 30.7305
      |   27.8508 27.8511 27.8513 27.8519 27.8525 27.8531 27.8537 27.8543 27.8548 27.8554 27.856 27.8566 27.8578 27.8595 27.8625 27.8804 27.9114 27.9769 28.2016 28.66 29.2059 29.8196 30.4829 31.1808 31.901
      |   29.5718 29.572 29.5723 29.5728 29.5733 29.5738 29.5744 29.5749 29.5754 29.5759 29.5765 29.577 29.578 29.5796 29.5822 29.5982 29.6258 29.6839 29.8821 30.2835 30.7601 31.2961 31.8774 32.4915 33.1284
      |   31.2285 31.2287 31.2289 31.2294 31.2298 31.2303 31.2308 31.2312 31.2317 31.2322 31.2327 31.2331 31.2341 31.2355 31.2379 31.2523 31.277 31.3291 31.5057 31.8614 32.2823 32.756 33.2709 33.817 34.3855
      |   32.8284 32.8286 32.8288 32.8293 32.8297 32.8301 32.8305 32.831 32.8314 32.8318 32.8322 32.8327 32.8335 32.8348 32.837 32.85 32.8724 32.9195 33.0784 33.3965 33.772 34.1946 34.655 35.1446 35.6562
      |   34.3782 34.3783 34.3785 34.3789 34.3793 34.3797 34.3801 34.3805 34.3809 34.3813 34.3816 34.382 34.3828 34.384 34.386 34.3979 34.4183 34.4612 34.6052 34.8921 35.2298 35.61 36.0247 36.4669 36.9303
      |   35.8832 35.8833 35.8835 35.8838 35.8842 35.8846 35.8849 35.8853 35.8856 35.886 35.8863 35.8867 35.8874 35.8885 35.8903 35.9013 35.92 35.9593 36.0907 36.3512 36.6572 37.0016 37.3777 37.7796 38.2018
      |   37.3481 37.3482 37.3484 37.3487 37.349 37.3494 37.3497 37.35 37.3504 37.3507 37.351 37.3514 37.352 37.353 37.3547 37.3648 37.3821 37.4183 37.5388 37.7769 38.0559 38.3698 38.7129 39.0801 39.4668
      |   38.777 38.7771 38.7773 38.7776 38.7779 38.7782 38.7785 38.7788 38.7791 38.7794 38.7797 38.78 38.7807 38.7816 38.7831 38.7925 38.8085 38.842 38.9532 39.1719 39.4277 39.7153 40.0299 40.3671 40.7229
      |   40.1734 40.1736 40.1737 40.174 40.1743 40.1746 40.1748 40.1751 40.1754 40.1757 40.176 40.1763 40.1768 40.1777 40.1792 40.1879 40.2028 40.2339 40.3369 40.5389 40.7745 41.0392 41.329 41.64 41.9687
      |   41.5405 41.5406 41.5407 41.541 41.5413 41.5415 41.5418 41.5421 41.5423 41.5426 41.5429 41.5431 41.5437 41.5445 41.5458 41.554 41.5679 41.5969 41.6928 41.88 42.098 42.3428 42.6108 42.8988 43.2035
      |   54.0647 54.0647 54.0648 54.065 54.0651 54.0653 54.0654 54.0656 54.0658 54.0659 54.0661 54.0662 54.0665 54.067 54.0678 54.0726 54.0808 54.0976 54.152 54.2554 54.3737 54.5055 54.6498 54.8053 54.971
      |   65.3877 65.3878 65.3878 65.388 65.3881 65.3882 65.3883 65.3884 65.3885 65.3886 65.3887 65.3888 65.389 65.3894 65.3899 65.3932 65.3988 65.4102 65.4468 65.5151 65.592 65.6771 65.7699 65.8698 65.9763
      | ] s*uPa
      k_TLU2=|
      | [
      |   13.9391 13.9416 13.9448 13.9512 13.9577 13.9642 13.9707 13.9773 13.984 13.9907 13.9974 14.0041 14.0178 14.0386 14.0742 14.3109 14.7946 16.1162 24.35 47.7184 60.1719 69.4118 77.1699 83.9998 90.1695
      |   14.8253 14.8277 14.8307 14.8367 14.8427 14.8488 14.855 14.8611 14.8673 14.8735 14.8798 14.8861 14.8988 14.9182 14.9512 15.1681 15.6015 16.7359 22.5568 40.204 52.9249 62.0901 69.7803 76.5816 82.7518
      |   15.6972 15.6994 15.7022 15.7079 15.7136 15.7193 15.725 15.7308 15.7366 15.7425 15.7483 15.7542 15.7661 15.7842 15.8149 16.0155 16.4092 17.4087 22.0259 35.1083 47.3353 56.273 63.7305 70.3606 76.4155
      |   16.5551 16.5573 16.5599 16.5652 16.5706 16.576 16.5814 16.5869 16.5923 16.5978 16.6033 16.6089 16.6201 16.637 16.6659 16.8524 17.2137 18.1104 21.9933 32.0591 43.0631 51.6942 58.8536 65.2262 71.081
      |   17.3997 17.4017 17.4042 17.4093 17.4143 17.4194 17.4246 17.4297 17.4349 17.4401 17.4453 17.4505 17.4611 17.4771 17.5042 17.6787 18.0128 18.8279 22.2078 30.3291 39.8783 48.0818 54.9381 61.0256 66.6351
      |   18.2313 18.2332 18.2356 18.2404 18.2452 18.2501 18.2549 18.2598 18.2647 18.2696 18.2746 18.2795 18.2895 18.3046 18.3303 18.4943 18.8054 19.5534 22.5621 29.382 37.5845 45.2309 51.7825 57.5935 62.9474
      |   22.2123 22.2138 22.2157 22.2195 22.2234 22.2272 22.2311 22.235 22.2389 22.2428 22.2467 22.2506 22.2585 22.2704 22.2905 22.4169 22.6488 23.1816 25.1622 29.0834 33.4651 38.1931 42.955 47.5107 51.8008
      |   25.9364 25.9377 25.9393 25.9425 25.9457 25.9489 25.9521 25.9553 25.9585 25.9618 25.965 25.9682 25.9748 25.9846 26.0012 26.1045 26.2906 26.7088 28.2215 31.1413 34.2397 37.4828 40.8497 44.2604 47.6337
      |   29.4481 29.4492 29.4505 29.4533 29.456 29.4588 29.4615 29.4643 29.467 29.4698 29.4725 29.4753 29.4809 29.4893 29.5034 29.5908 29.7465 30.0913 31.3189 33.6811 36.1618 38.6932 41.2846 43.9311 46.6062
      |   32.7824 32.7833 32.7845 32.7869 32.7893 32.7917 32.7941 32.7965 32.7989 32.8013 32.8037 32.8062 32.811 32.8183 32.8306 32.9064 33.0402 33.3334 34.3647 36.3504 38.4417 40.5559 42.6906 44.8551 47.049
      |   35.967 35.9679 35.9689 35.971 35.9732 35.9753 35.9774 35.9796 35.9817 35.9838 35.986 35.9881 35.9925 35.9989 36.0098 36.0767 36.1941 36.4489 37.3368 39.0473 40.861 42.6938 44.5307 46.3782 48.2427
      |   39.0242 39.025 39.0259 39.0278 39.0297 39.0317 39.0336 39.0355 39.0374 39.0393 39.0413 39.0432 39.0471 39.0529 39.0626 39.1225 39.227 39.4524 40.2307 41.7306 43.3323 44.9566 46.581 48.2059 49.8373
      |   41.9719 41.9726 41.9734 41.9752 41.9769 41.9786 41.9804 41.9821 41.9839 41.9856 41.9874 41.9891 41.9926 41.9979 42.0068 42.0609 42.1551 42.357 43.0492 44.3824 45.8152 47.2758 48.7378 50.1965 51.6553
      |   44.8247 44.8253 44.8261 44.8277 44.8293 44.8309 44.8325 44.8341 44.8357 44.8373 44.8389 44.8405 44.8437 44.8485 44.8566 44.9061 44.9918 45.1747 45.7973 46.9952 48.2899 49.6168 50.9485 52.2766 53.6018
      |   47.5948 47.5953 47.5961 47.5976 47.599 47.6005 47.602 47.6034 47.6049 47.6064 47.6079 47.6094 47.6123 47.6168 47.6242 47.6698 47.7484 47.9155 48.4809 49.567 50.7462 51.9612 53.1847 54.4062 55.6239
      |   50.2923 50.2928 50.2935 50.2948 50.2962 50.2976 50.2989 50.3003 50.3017 50.3031 50.3044 50.3058 50.3086 50.3127 50.3196 50.3618 50.4344 50.5882 51.1057 52.0979 53.1792 54.2987 55.4303 56.5622 57.6906
      |   52.9257 52.9262 52.9269 52.9281 52.9294 52.9307 52.9319 52.9332 52.9345 52.9358 52.9371 52.9383 52.9409 52.9448 52.9512 52.9905 53.058 53.2004 53.6773 54.5897 55.5868 56.6238 57.6759 58.7307 59.7832
      |   55.5024 55.5029 55.5034 55.5046 55.5058 55.507 55.5082 55.5094 55.5106 55.5118 55.513 55.5142 55.5166 55.5202 55.5263 55.563 55.6261 55.7587 56.2006 57.0444 57.9686 58.9334 59.9158 60.9033 61.89
      |   58.0285 58.0289 58.0295 58.0306 58.0317 58.0329 58.034 58.0351 58.0362 58.0374 58.0385 58.0396 58.0419 58.0453 58.051 58.0855 58.1446 58.2687 58.6804 59.4645 60.3248 61.2261 62.1468 63.0747 64.0035
      |   60.5094 60.5098 60.5104 60.5114 60.5125 60.5135 60.5146 60.5157 60.5167 60.5178 60.5189 60.5199 60.5221 60.5253 60.5306 60.5632 60.6189 60.7354 61.1206 61.8525 62.6566 63.5013 64.367 65.2418 66.119
      |   62.9498 62.9502 62.9507 62.9517 62.9527 62.9537 62.9547 62.9557 62.9567 62.9577 62.9588 62.9598 62.9618 62.9648 62.9699 63.0007 63.0533 63.1632 63.525 64.2108 64.9649 65.7593 66.5756 67.4024 68.2333
      |   65.3537 65.3541 65.3546 65.3556 65.3565 65.3575 65.3584 65.3594 65.3603 65.3613 65.3622 65.3632 65.3651 65.368 65.3728 65.402 65.4519 65.5558 65.8969 66.5418 67.2513 68.0003 68.772 69.5555 70.3443
      |   88.0086 88.0089 88.0092 88.0098 88.0104 88.0111 88.0117 88.0124 88.013 88.0136 88.0143 88.0149 88.0162 88.0181 88.0213 88.0406 88.0734 88.1407 88.3566 88.7555 89.1929 89.6591 90.1466 90.6495 91.1636
      |   109.301 109.301 109.302 109.302 109.303 109.303 109.304 109.304 109.305 109.305 109.305 109.306 109.307 109.308 109.311 109.325 109.35 109.399 109.557 109.843 110.153 110.485 110.832 111.193 111.565
      | ] mW/(K*m)
      beta_TLU2=|
      | [
      |   0.000999942 0.00499856 0.00999424 0.019977 0.0299481 0.0399077 0.0498557 0.0597921 0.0697169 0.0796301 0.0895315 0.0994213 0.119166 0.148694 0.197672 0.485202 0.939079 1.74175 3.21852 14.5551 40.7994 70.0982 100.32 130.872 161.527
      |   0.000999953 0.00499883 0.00999532 0.0199813 0.0299578 0.039925 0.0498827 0.0598311 0.06977 0.0796995 0.0896195 0.0995301 0.119323 0.148941 0.198114 0.488094 0.951588 1.80052 3.74577 10.3273 29.4662 54.2365 81.1248 109.027 137.464
      |   0.000999962 0.00499904 0.00999617 0.0199847 0.0299655 0.0399386 0.0499041 0.0598618 0.0698119 0.0797543 0.089689 0.0996159 0.119447 0.149135 0.198461 0.490338 0.961089 1.84299 4.07288 9.2541 23.0773 43.5243 67.0627 92.2475 118.402
      |   0.000999968 0.00499921 0.00999685 0.0199874 0.0299716 0.0399495 0.0499211 0.0598864 0.0698454 0.0797981 0.0897445 0.0996846 0.119546 0.14929 0.198738 0.492112 0.968478 1.87488 4.29554 9.12165 19.7101 36.49 56.9418 79.5087 103.415
      |   0.000999974 0.00499935 0.0099974 0.0199896 0.0299766 0.0399584 0.049935 0.0599064 0.0698726 0.0798336 0.0897895 0.0997401 0.119626 0.149416 0.198962 0.493534 0.974331 1.89949 4.4562 9.23686 17.9884 31.9473 49.7235 69.9071 91.6925
      |   0.000999979 0.00499946 0.00999785 0.0199914 0.0299807 0.0399656 0.0499463 0.0599227 0.0698949 0.0798627 0.0898263 0.0997856 0.119691 0.149518 0.199144 0.494689 0.97904 1.91891 4.57685 9.40373 17.1049 29.0338 44.5848 62.6809 82.5405
      |   0.000999992 0.0049998 0.00999921 0.0199968 0.0299929 0.0399874 0.0499803 0.0599717 0.0699615 0.0799497 0.0899364 0.0999215 0.119887 0.149824 0.199688 0.498099 0.992713 1.97351 4.89126 10.0266 16.2093 24.0824 33.8923 45.5732 58.9199
      |   0.000999998 0.00499995 0.00999982 0.0199993 0.0299984 0.0399971 0.0499955 0.0599935 0.0699912 0.0799885 0.0899855 0.0999822 0.119974 0.14996 0.199931 0.4996 0.998624 1.99633 5.01265 10.3006 16.2398 23.135 31.1669 40.3929 50.7853
      |   0.001 0.00500003 0.0100001 0.0200005 0.0300011 0.0400019 0.050003 0.0600043 0.0700059 0.0800077 0.0900098 0.100012 0.120017 0.150028 0.20005 0.500333 1.00149 2.00718 5.06781 10.422 16.2732 22.7909 30.0876 38.22 47.1991
      |   0.001 0.00500007 0.0100003 0.0200011 0.0300025 0.0400044 0.0500069 0.0600099 0.0700135 0.0800176 0.0900223 0.100028 0.12004 0.150062 0.200111 0.500711 1.00295 2.01265 5.09439 10.4746 16.2707 22.5865 29.4948 37.0382 45.2335
      |   0.001 0.00500009 0.0100004 0.0200014 0.0300032 0.0400057 0.0500089 0.0600128 0.0700175 0.0800229 0.0900289 0.100036 0.120052 0.150081 0.200144 0.500909 1.00371 2.01543 5.10703 10.4936 16.2448 22.4285 29.0935 36.2708 43.9756
      |   0.001 0.0050001 0.0100004 0.0200016 0.0300036 0.0400064 0.05001 0.0600143 0.0700195 0.0800255 0.0900323 0.10004 0.120057 0.15009 0.20016 0.501008 1.00409 2.01677 5.11233 10.495 16.2063 22.2922 28.7865 35.7117 43.0802
      |   0.001 0.0050001 0.0100004 0.0200017 0.0300038 0.0400067 0.0500104 0.060015 0.0700205 0.0800267 0.0900338 0.100042 0.12006 0.150094 0.200167 0.501052 1.00425 2.0173 5.11361 10.4872 16.1619 22.1697 28.5347 35.2732 42.3947
      |   0.001 0.00500011 0.0100004 0.0200017 0.0300038 0.0400068 0.0500106 0.0600152 0.0700207 0.0800271 0.0900343 0.100042 0.120061 0.150095 0.20017 0.501064 1.00429 2.01738 5.11263 10.4745 16.1153 22.0579 28.3195 34.9122 41.843
      |   0.001 0.00500011 0.0100004 0.0200017 0.0300038 0.0400067 0.0500105 0.0600152 0.0700206 0.0800269 0.0900341 0.100042 0.120061 0.150095 0.200169 0.501057 1.00425 2.01718 5.11039 10.4594 16.0688 21.9552 28.1311 34.6053 41.3831
      |   0.001 0.0050001 0.0100004 0.0200017 0.0300037 0.0400066 0.0500103 0.0600149 0.0700203 0.0800265 0.0900335 0.100041 0.12006 0.150093 0.200166 0.501039 1.00417 2.01682 5.10744 10.4432 16.0236 21.8606 27.9635 34.3386 40.9898
      |   0.001 0.0050001 0.0100004 0.0200016 0.0300036 0.0400065 0.0500101 0.0600146 0.0700198 0.0800259 0.0900328 0.10004 0.120058 0.150091 0.200162 0.501014 1.00407 2.01638 5.10414 10.4268 15.9802 21.7733 27.8128 34.1032 40.6473
      |   0.001 0.0050001 0.0100004 0.0200016 0.0300035 0.0400063 0.0500098 0.0600142 0.0700193 0.0800252 0.0900319 0.100039 0.120057 0.150089 0.200157 0.500986 1.00395 2.01589 5.10069 10.4107 15.9391 21.6926 27.6762 33.8929 40.3447
      |   0.001 0.0050001 0.0100004 0.0200015 0.0300034 0.0400061 0.0500095 0.0600137 0.0700187 0.0800244 0.0900309 0.100038 0.120055 0.150086 0.200153 0.500956 1.00383 2.01538 5.09722 10.395 15.9002 21.6179 27.5515 33.7033 40.0744
      |   0.001 0.00500009 0.0100004 0.0200015 0.0300033 0.0400059 0.0500092 0.0600133 0.0700181 0.0800236 0.0900299 0.100037 0.120053 0.150083 0.200148 0.500925 1.00371 2.01487 5.0938 10.3799 15.8637 21.5487 27.4373 33.5312 39.8309
      |   0.001 0.00500009 0.0100004 0.0200014 0.0300032 0.0400057 0.0500089 0.0600129 0.0700175 0.0800229 0.090029 0.100036 0.120051 0.15008 0.200143 0.500895 1.00358 2.01437 5.09048 10.3656 15.8293 21.4843 27.3323 33.374 39.6098
      |   0.001 0.00500009 0.0100003 0.0200014 0.0300031 0.0400055 0.0500086 0.0600124 0.0700169 0.0800221 0.090028 0.100035 0.12005 0.150078 0.200138 0.500865 1.00346 2.01388 5.08728 10.352 15.7971 21.4245 27.2352 33.2297 39.408
      |   0.001 0.00500006 0.0100003 0.020001 0.0300023 0.040004 0.0500063 0.060009 0.0700123 0.080016 0.0900203 0.100025 0.120036 0.150056 0.2001 0.500626 1.00251 2.01002 5.06265 10.2506 15.5634 21.0005 26.5612 32.2445 38.0494
      |   0.001 0.00500005 0.0100002 0.0200008 0.0300017 0.0400031 0.0500048 0.0600069 0.0700094 0.0800123 0.0900155 0.100019 0.120028 0.150043 0.200077 0.500478 1.00191 2.00765 5.04777 10.1907 15.4281 20.7593 26.1834 31.6997 37.3074
      | ] MPa
      alpha_TLU2=|
      | [
      |   0.00666787 0.00667271 0.00667876 0.00669089 0.00670305 0.00671525 0.00672749 0.00673976 0.00675206 0.0067644 0.00677678 0.00678919 0.00681412 0.00685179 0.00691531 0.00731685 0.00807384 0.0100186 0.0227829 0.0193522 0.0105807 0.0076844 0.00622882 0.00533765 0.00472794
      |   0.00625095 0.00625475 0.0062595 0.00626903 0.00627857 0.00628814 0.00629772 0.00630733 0.00631696 0.00632662 0.00633629 0.00634599 0.00636544 0.00639479 0.00644415 0.00675235 0.00731604 0.00866732 0.0152659 0.0192717 0.011494 0.00818787 0.00652667 0.00552549 0.00485096
      |   0.00588311 0.00588614 0.00588993 0.00589751 0.00590511 0.00591273 0.00592035 0.00592799 0.00593565 0.00594331 0.00595099 0.00595869 0.00597411 0.00599735 0.00603636 0.00627767 0.00670918 0.00769477 0.011767 0.0162116 0.0116594 0.008463 0.00672213 0.00565673 0.00493839
      |   0.00555617 0.00555861 0.00556167 0.00556779 0.00557392 0.00558005 0.0055862 0.00559235 0.00559851 0.00560468 0.00561086 0.00561705 0.00562944 0.0056481 0.00567937 0.00587141 0.00620899 0.00695322 0.00971437 0.013198 0.0110941 0.00846206 0.00678841 0.00571713 0.00498243
      |   0.00526366 0.00526565 0.00526814 0.00527314 0.00527813 0.00528313 0.00528814 0.00529315 0.00529817 0.00530319 0.00530822 0.00531325 0.00532333 0.00533849 0.00536386 0.00551881 0.00578754 0.0063644 0.00835021 0.0109416 0.0101405 0.00821375 0.00672515 0.0057025 0.00497969
      |   0.00500041 0.00500205 0.00500411 0.00500822 0.00501233 0.00501645 0.00502056 0.00502469 0.00502881 0.00503294 0.00503707 0.00504121 0.00504949 0.00506193 0.00508273 0.00520921 0.00542625 0.00588259 0.00736985 0.00930984 0.00911629 0.00779577 0.00655315 0.00561931 0.00493193
      |   0.00400017 0.00400087 0.00400173 0.00400347 0.0040052 0.00400694 0.00400867 0.00401041 0.00401214 0.00401388 0.00401561 0.00401735 0.00402082 0.00402602 0.0040347 0.00408675 0.00417337 0.00434539 0.00483362 0.00542968 0.00561413 0.00543555 0.00507088 0.00466062 0.00427229
      |   0.00333342 0.00333375 0.00333416 0.00333499 0.00333582 0.00333664 0.00333747 0.0033383 0.00333912 0.00333995 0.00334077 0.0033416 0.00334325 0.00334572 0.00334983 0.00337436 0.00341462 0.00349259 0.00370157 0.00394325 0.00403455 0.00399405 0.00386383 0.00368634 0.0034922
      |   0.00285719 0.00285735 0.00285757 0.00285799 0.00285841 0.00285883 0.00285926 0.00285968 0.0028601 0.00286052 0.00286094 0.00286136 0.0028622 0.00286346 0.00286556 0.002878 0.00289824 0.00293684 0.00303661 0.00314554 0.00318344 0.00316092 0.00309409 0.00299911 0.0028892
      |   0.00250002 0.00250011 0.00250022 0.00250045 0.00250067 0.00250089 0.00250111 0.00250133 0.00250156 0.00250178 0.002502 0.00250222 0.00250266 0.00250332 0.00250442 0.00251093 0.00252145 0.00254123 0.00259054 0.0026397 0.00265066 0.00262981 0.00258493 0.0025236 0.00245222
      |   0.00222223 0.00222228 0.00222234 0.00222245 0.00222257 0.00222269 0.0022228 0.00222292 0.00222303 0.00222315 0.00222327 0.00222338 0.00222361 0.00222396 0.00222453 0.0022279 0.00223331 0.0022433 0.00226689 0.0022862 0.00228329 0.00226213 0.002227 0.00218192 0.00213035
      |   0.00200001 0.00200003 0.00200006 0.00200011 0.00200017 0.00200023 0.00200028 0.00200034 0.0020004 0.00200045 0.00200051 0.00200057 0.00200068 0.00200085 0.00200112 0.00200275 0.00200533 0.00200992 0.00201958 0.00202306 0.00201292 0.0019917 0.00196196 0.001926 0.00188585
      |   0.00181818 0.00181819 0.0018182 0.00181823 0.00181825 0.00181827 0.00181829 0.00181832 0.00181834 0.00181836 0.00181838 0.00181841 0.00181845 0.00181852 0.00181862 0.00181925 0.00182019 0.00182171 0.00182353 0.00181837 0.00180453 0.00178371 0.0017575 0.00172733 0.00169442
      |   0.00166667 0.00166667 0.00166667 0.00166667 0.00166667 0.00166668 0.00166668 0.00166668 0.00166668 0.00166668 0.00166669 0.00166669 0.00166669 0.0016667 0.00166671 0.00166674 0.00166673 0.00166646 0.00166379 0.00165388 0.00163831 0.00161821 0.00159463 0.00156849 0.00154056
      |   0.00153846 0.00153846 0.00153845 0.00153844 0.00153843 0.00153842 0.00153841 0.0015384 0.00153839 0.00153838 0.00153837 0.00153836 0.00153834 0.00153831 0.00153826 0.00153795 0.00153737 0.00153605 0.00153081 0.00151839 0.00150218 0.001483 0.00146154 0.0014384 0.00141411
      |   0.00142857 0.00142856 0.00142855 0.00142854 0.00142852 0.0014285 0.00142849 0.00142847 0.00142845 0.00142844 0.00142842 0.0014284 0.00142837 0.00142832 0.00142823 0.00142771 0.00142681 0.00142488 0.00141821 0.00140457 0.00138837 0.00137019 0.00135051 0.00132975 0.00130824
      |   0.00133333 0.00133332 0.00133331 0.00133329 0.00133327 0.00133325 0.00133323 0.00133321 0.00133319 0.00133317 0.00133314 0.00133312 0.00133308 0.00133302 0.00133291 0.00133227 0.00133119 0.00132892 0.00132152 0.00130743 0.0012916 0.00127445 0.00125631 0.00123749 0.00121821
      |   0.00125 0.00124999 0.00124998 0.00124995 0.00124993 0.00124991 0.00124988 0.00124986 0.00124984 0.00124982 0.00124979 0.00124977 0.00124972 0.00124965 0.00124954 0.00124884 0.00124765 0.00124523 0.00123751 0.00122343 0.00120817 0.00119203 0.00117526 0.00115806 0.00114061
      |   0.00117647 0.00117646 0.00117645 0.00117642 0.0011764 0.00117637 0.00117635 0.00117633 0.0011763 0.00117628 0.00117625 0.00117623 0.00117618 0.00117611 0.00117599 0.00117526 0.00117404 0.00117155 0.00116378 0.00114999 0.0011354 0.00112024 0.00110468 0.00108888 0.00107296
      |   0.00111111 0.0011111 0.00111109 0.00111106 0.00111104 0.00111101 0.00111099 0.00111097 0.00111094 0.00111092 0.00111089 0.00111087 0.00111082 0.00111075 0.00111063 0.0011099 0.00110867 0.00110619 0.00109853 0.00108518 0.0010713 0.00105707 0.0010426 0.00102802 0.00101341
      |   0.00105263 0.00105262 0.00105261 0.00105258 0.00105256 0.00105254 0.00105251 0.00105249 0.00105246 0.00105244 0.00105242 0.00105239 0.00105234 0.00105227 0.00105215 0.00105143 0.00105023 0.00104779 0.00104034 0.00102752 0.00101437 0.001001 0.000987519 0.000974008 0.000960528
      |   0.000999998 0.000999988 0.000999977 0.000999953 0.00099993 0.000999907 0.000999883 0.00099986 0.000999837 0.000999813 0.00099979 0.000999767 0.00099972 0.00099965 0.000999533 0.000998832 0.000997658 0.000995296 0.000988106 0.000975864 0.000963414 0.000950858 0.00093827 0.00092571 0.000913225
      |   0.000666665 0.000666659 0.000666652 0.000666637 0.000666622 0.000666607 0.000666593 0.000666578 0.000666563 0.000666548 0.000666533 0.000666518 0.000666489 0.000666444 0.00066637 0.000665926 0.000665186 0.000663707 0.000659292 0.000652008 0.000644829 0.000637765 0.000630822 0.000624005 0.000617313
      |   0.000499999 0.000499995 0.000499991 0.000499981 0.000499972 0.000499963 0.000499953 0.000499944 0.000499935 0.000499925 0.000499916 0.000499906 0.000499888 0.00049986 0.000499813 0.000499533 0.000499066 0.000498136 0.000495362 0.000490801 0.000486321 0.000481921 0.000477602 0.000473363 0.000469203
      | ] 1/K
  PS-Simulink Converter{1..10} (10 alike) : nesl_utility/PS-Simulink Converter  PhysicalDomain=network_engine_domain  SubClassName=ps_output  LeftPortType=input  RightPortType=output  PseudoPeriodic=off  Frequencies=[]  VectorFormat=inherit  Unit=inherit  AffineConversion=off
  Pressurant Mass Flow Rate : Scope
      settings: ActiveDisplayYMinimum=0.031327551586104771  ActiveDisplayYMaximum=0.20523704127947895  DataLoggingVariableName=ScopeData14
  Pressure & Temperature Sensor (TL){,1..3} (4 alike) : fl_lib/Thermal Liquid/Sensors/Pressure & Temperature Sensor (TL)  reference=foundation.enum.MeasurementReference.absolute  pressure=true  pressure_spec=foundation.enum.PressureMeasementSpec.Absolute  temperature=false
      settings: InternalSimscapePortConfiguration="{\"Bottom\":[],\"Left\":[{\"id\":\"A\",\"label\":\"A\",\"type\":\"foundation.thermal_liquid.thermal_liquid\"}],\"Right\":[{\"id\":\"Pa\",\"label\":\"Pa\",\"type\":\"output\"}],\"Top\":[]}"
  Pressure Source (TL) : fl_lib/Thermal Liquid/Sources/Pressure Source (TL)  source_type=foundation.enum.constant_controlled.controlled  pressure_differential=0 MPa  power_spec=foundation.enum.power_spec.isentropic  area=0.01 m^2
      settings: InternalSimscapePortConfiguration="{\"Bottom\":[],\"Left\":[{\"id\":\"A\",\"label\":\"A\",\"type\":\"foundation.thermal_liquid.thermal_liquid\"},{\"id\":\"P\",\"label\":\"P\",\"type\":\"input\"}],\"Right\":[{\"id\":\"B\",\"label\":\"B\",\"type\":\"foundation.thermal_liquid.thermal_liquid\"}],\"Top\":[]}"
  Pressure Source (TL)1 : fl_lib/Thermal Liquid/Sources/Pressure Source (TL)  source_type=foundation.enum.constant_controlled.controlled  pressure_differential=0 MPa  power_spec=foundation.enum.power_spec.isentropic  area=0.01 m^2
      settings: InternalSimscapePortConfiguration="{\"Bottom\":[],\"Left\":[{\"id\":\"A\",\"label\":\"A\",\"type\":\"foundation.thermal_liquid.thermal_liquid\"},{\"id\":\"P\",\"label\":\"P\",\"type\":\"input\"}],\"Right\":[{\"id\":\"B\",\"label\":\"B\",\"type\":\"foundation.thermal_liquid.thermal_liquid\"}],\"Top\":[]}"
  Reservoir (TL) : fl_lib/Thermal Liquid/Elements/Reservoir (TL)  pressure_spec=foundation.enum.pressure_spec.atmospheric  reservoir_pressure=0.101325 MPa  reservoir_temperature=293.15 K  area=0.01 m^2
  Reservoir (TL)1 : fl_lib/Thermal Liquid/Elements/Reservoir (TL)  pressure_spec=foundation.enum.pressure_spec.atmospheric  reservoir_pressure=0.101325 MPa  reservoir_temperature=100 K  area=0.01 m^2
  Simulink-PS Converter{1..4} (4 alike) : nesl_utility/Simulink-PS Converter  PhysicalDomain=network_engine_domain  SubClassName=ps_input  LeftPortType=input  RightPortType=output  PseudoPeriodic=off  Frequencies=[]  NoiseDistribution=none  NoiseParameters=[]  Unit=1  AffineConversion=off  FilteringAndDerivatives=provide  SimscapeFilterOrder=1  InputFilterTimeConstant=0.001  UdotUserProvided=0
  Subsystem Reference1 : Subsystem  ReferencedSubsystem=PT  max_press=5000  lower_val=4  upper_val=20
  Temperature Sensor2 : fl_lib/Thermal/Thermal Sensors/Temperature Sensor  temperature_measure=foundation.enum.MeasurementReference.difference
  Thermal Ref3 (0K) : fl_lib/Thermal/Thermal Elements/Thermal Reference
  Thermodynamic Properties Sensor (TL) : fl_lib/Thermal Liquid/Sensors/Thermodynamic Properties Sensor (TL)  internal_energy=false  density=true  specific_heat=false
      settings: InternalSimscapePortConfiguration="{\"Bottom\":[],\"Left\":[{\"id\":\"A\",\"label\":\"A\",\"type\":\"foundation.thermal_liquid.thermal_liquid\"}],\"Right\":[{\"id\":\"RHO\",\"label\":\"ρ\",\"type\":\"output\"}],\"Top\":[]}"
  Thermodynamic Properties Sensor (TL)1 : fl_lib/Thermal Liquid/Sensors/Thermodynamic Properties Sensor (TL)  internal_energy=false  density=true  specific_heat=false
      settings: InternalSimscapePortConfiguration="{\"Bottom\":[],\"Left\":[{\"id\":\"A\",\"label\":\"A\",\"type\":\"foundation.thermal_liquid.thermal_liquid\"}],\"Right\":[{\"id\":\"RHO\",\"label\":\"ρ\",\"type\":\"output\"}],\"Top\":[]}"
  Thrust : Scope
      settings: ActiveDisplayYMinimum=-35.792502098201048  ActiveDisplayYMaximum=322.91167155982083  DataLoggingVariableName=ScopeData21
  wires:
  Subsystem Reference1/1 -> COPV PT/1
  PS-Simulink Converter4/1 -> N2 Temp COPV/1
  PS-Simulink Converter9/1 -> Pressurant Mass Flow Rate/1
  PS-Simulink Converter5/1 -> MATLAB Function/1(mdot_ox)
  PS-Simulink Converter1/1 -> MATLAB Function/2(mdot_fuel)
  Constant/1 -> MATLAB Function/4(Cf)
  Constant1/1 -> MATLAB Function/3(eta_cstar)
  MATLAB Function/2(Pc) -> Simulink-PS Converter4/1, Simulink-PS Converter1/1, Gain/1
  Gain/1 -> Chamber Pressure/1
  Gain1/1 -> Thrust/1
  MATLAB Function/1(thrust) -> Gain1/1
  PS-Simulink Converter2/1 -> MATLAB Function1/2(rho_ox)
  PS-Simulink Converter7/1 -> MATLAB Function1/4(rho_fuel)
  PS-Simulink Converter3/1 -> MATLAB Function2/1(P_up)
  PS-Simulink Converter6/1 -> MATLAB Function2/2(P_down)
  MATLAB Function2/1(dP) -> MATLAB Function1/3(dP_ox)
  PS-Simulink Converter8/1 -> MATLAB Function3/1(P_up)
  PS-Simulink Converter10/1 -> MATLAB Function3/2(P_down)
  MATLAB Function3/1(dP) -> MATLAB Function1/5(dP_fuel)
  MATLAB Function1/1(CdA_ox_des) -> MATLAB Function4/1(CdA_ox_des)
  MATLAB Function1/2(CdA_fuel_des) -> MATLAB Function4/2(CdA_fuel_des)
  MATLAB Function4/1(opening_ox) -> Simulink-PS Converter2/1
  MATLAB Function4/2(opening_fuel) -> Simulink-PS Converter3/1
  Clock/1 -> 1-D Lookup Table/1
  1-D Lookup Table/1 -> MATLAB Function1/1(F_cmd)
  connections:
  LBB/RConn1 -- Lox Tank/LConn1
  FBB/RConn1 -- Fuel Tank/LConn1
  LBB/LConn1 -- Subsystem Reference1/LConn1 -- FBB/LConn1 -- Nitrogen Properties/RConn1 -- Mass & Energy Flow Rate Sensor (G)/RConn1 -- COPV Leakage/RConn1
  PS-Simulink Converter9/LConn1 -- Mass & Energy Flow Rate Sensor (G)/RConn2
  COPV/RConn1 -- Mass & Energy Flow Rate Sensor (G)/LConn1
  Thermal Ref3 (0K)/LConn1 -- Temperature Sensor2/RConn1
  Temperature Sensor2/LConn1 -- COPV/LConn2
  PS-Simulink Converter4/LConn1 -- Temperature Sensor2/RConn2
  Mass & Energy Flow Rate Sensor (TL)1/RConn1 -- Pressure Source (TL)/RConn1
  Local Restriction (TL)/LConn1 -- Pressure Source (TL)/LConn1
  Reservoir (TL)/LConn1 -- Local Restriction (TL)/RConn1
  Simulink-PS Converter4/RConn1 -- Pressure Source (TL)/LConn2
  PS-Simulink Converter5/LConn1 -- Mass & Energy Flow Rate Sensor (TL)/RConn2
  PS-Simulink Converter1/LConn1 -- Mass & Energy Flow Rate Sensor (TL)1/RConn2
  Simulink-PS Converter1/RConn1 -- Pressure Source (TL)1/LConn2
  Local Restriction (TL)1/LConn1 -- Pressure Source (TL)1/LConn1
  Reservoir (TL)1/LConn1 -- Local Restriction (TL)1/RConn1
  Pressure Source (TL)1/RConn1 -- Mass & Energy Flow Rate Sensor (TL)/RConn1
  2-Way Directional Valve (TL)/RConn2 -- Mass & Energy Flow Rate Sensor (TL)1/LConn1 -- Pressure & Temperature Sensor (TL)3/LConn1
  2-Way Directional Valve (TL)1/RConn2 -- Pressure & Temperature Sensor (TL)1/LConn1 -- Mass & Energy Flow Rate Sensor (TL)/LConn1
  Simulink-PS Converter2/RConn1 -- 2-Way Directional Valve (TL)1/RConn1
  Simulink-PS Converter3/RConn1 -- 2-Way Directional Valve (TL)/RConn1
  Fuel Tank/RConn1 -- 2-Way Directional Valve (TL)/LConn1 -- Thermodynamic Properties Sensor (TL)1/LConn1 -- Pressure & Temperature Sensor (TL)2/LConn1
  Lox Tank/RConn1 -- Pressure & Temperature Sensor (TL)/LConn1 -- 2-Way Directional Valve (TL)1/LConn1 -- Thermodynamic Properties Sensor (TL)/LConn1
  Thermodynamic Properties Sensor (TL)/RConn1 -- PS-Simulink Converter2/LConn1
  Pressure & Temperature Sensor (TL)/RConn1 -- PS-Simulink Converter3/LConn1
  Pressure & Temperature Sensor (TL)1/RConn1 -- PS-Simulink Converter6/LConn1
  Pressure & Temperature Sensor (TL)2/RConn1 -- PS-Simulink Converter8/LConn1
  Thermodynamic Properties Sensor (TL)1/RConn1 -- PS-Simulink Converter7/LConn1
  Pressure & Temperature Sensor (TL)3/RConn1 -- PS-Simulink Converter10/LConn1
